simulink model "QET_KV"  (R2015b)
settings: Solver=ode4  SolverMode=SingleTasking  StartTime=0.0  StopTime=inf  FixedStep=Ts  RelTol=1e-3
values from neighbouring files (symbols this model uses):
  F_M_Direction = [1 1 1 -1 -1 -1]    [Config_StepperMotor.m]
  NanoCal7342 = [-0.945276141167 14.673559188843 0.251662999392 -14.892200469971 -0.854624807835 0.034513175488 ... (first row only)    [NanoCalibration.m]
  Resolution = (360/200 * 1/64)    (= 0.028125)    [Config_StepperMotor.m]
undefined symbols (not defined in the file or in its folder): AnalogPos_to_deg, anVE, anVE_GBC_Kbi, anVE_GBC_Kbp, anVE_K_int, anVE_Position_Gain_inv, anVE_Saturation, B, Chirp_Amplitude, Chirp_Freq_Max, Chirp_Freq_Min, Chirp_Period, Chirp_Time_Start, Chirp_Type, delay, Delta, DO_DG409_A0, DO_DG409_A1, Driver_Type, HIL, K, K_gyro, Kd, Kp, lambda, mag, Pos_Final, Pos_Init, Pos_Threshold, PSoC_Freq, qc_get_step_size, Stabilization_Period, Test_type, Times, Torque_Threshold, Ts, Ts_loop, VE_Platform, VE_Type
libraries: quarc_library x22, simulink x13, dspsigops x1
(part 3 of 3)

== matlab function QET_KV/Stability Check and Control/Initial and Final Condition Control/MATLAB Function ==
  data: sw output; sw_Sequence output; Clock input; Times input; Pos_Init input; Pos_out output; Pos_in input; is_stable input; Pos_Final input
function [sw,sw_Sequence,Pos_out] = fcn(Clock,Times,Pos_Init,Pos_in,is_stable,Pos_Final)
%#codegen


sw = 1;
Pos_out = 0;

%%
% Starting Up
if (Clock<Times(1))
    sw = 1;
    sw_Sequence = 1;
    Pos_out = 0;
% Initial Condition
elseif (Clock<Times(2))
    sw = 1;
    sw_Sequence = 2;
    Pos_out = Pos_Init;
% Stability Test
elseif (Clock<Times(3))&&(is_stable)
    sw = 2;
    sw_Sequence = 3;
    %Pos_out = Pos_in;
    Pos_out = Pos_Final;
% Final Condition
else
    sw = 1;
    sw_Sequence = 4;
    Pos_out = Pos_Final;
end

== matlab function QET_KV/PSoC Comm/MATLAB Function1 ==
  data: K input; X input; cmd output uint8; clock input; en output
function [cmd, en] = fcn(K,X,clock)
%#codegen


%cmd = cast('     ','uint8');
sum_ = 0;
cmd = uint8(zeros(1,6));
if (clock == 0.5)
    en = 1;
%    cmd = cast('Kabcd','uint8');
    cmd(1) = uint8('K');
    cmd(2:5) = typecast(single(K),'uint8');
    
    sum_ = mod(sum(cmd),256);
    cmd(6) = 255-sum_;
    
elseif (clock == 1)
    en = 1;
    cmd(1) = uint8('X');
    cmd(2:5) = typecast(single(X),'uint8');
    
    sum_ = mod(sum(cmd),256);
    cmd(6) = 255-sum_;
elseif (clock == 4)
    en = 1;
    cmd(1) = uint8('X');
    cmd(2:5) = typecast(single(0),'uint8');
    
    sum_ = mod(sum(cmd),256);
    cmd(6) = 255-sum_;
else
    en = 0;
end

== matlab function QET_KV/Stability Check and Control/Stability Check/MATLAB Function ==
  data: is_stable output; Clock input; Times input; Pos input; Pos_LPF input; Pos_Init input; Stop_PosThreshold input; stop_sim output; stop_sim_final output; Torque_Threshold input; Torque_LPF input; Pos_Threshold input; Pos_Random input; Stab_Period input; is_saturated input
function [is_stable,stop_sim,stop_sim_final]   = fcn(Clock, Times, Pos, Pos_LPF, Pos_Init, Stop_PosThreshold, Torque_Threshold, Torque_LPF, Pos_Threshold, Pos_Random,Stab_Period,is_saturated)
%#codegen
%% Initialization
persistent var_is_stable clock_stop;
if isempty(var_is_stable)
    var_is_stable = 1;
end
if isempty(clock_stop)
    clock_stop = 10;
end
%Pos_Threshold = Pos_Init * 1.25;

%% Define if is NOT stable

%Based on position threshold during uncoupled test
%Between times(1) and times (3)
%if ((Clock >= Times(2))...
    %&&(Clock < Times(3))...
if ((Clock >= Times(1))...
    &&(abs(Pos) >= Pos_Threshold)...
    &&(var_is_stable==1))
    var_is_stable = 0;
    clock_stop = Clock+Stab_Period;
end

%Based on Torque Threshold
if ((Clock>=Times(1))...
    &&(Torque_LPF >= Torque_Threshold)...
    &&(var_is_stable==1))
    var_is_stable = 0;
    clock_stop = Clock+Stab_Period;
end

%If there is saturation
if ((Clock>=Times(1))...
    &&(is_saturated > 0.5)...
    &&(var_is_stable==1))
    var_is_stable = 0;
    clock_stop = Clock+Stab_Period;
end

%% Stop simulation rules
stop_sim = 0;

if (var_is_stable==1)
    if (Clock<Times(3))
        Pos_Abs_Error = abs(Pos_LPF - 0);
    else
        Pos_Abs_Error = abs(Pos_LPF - Pos_Random)*.75;
    end
else
    Pos_Abs_Error = abs(Pos_LPF - Pos_Random)*.75;
end

% If it is Stable
if ((var_is_stable == 1)...
    &&(Clock>Times(3)+1.5)...
    &&(Pos_Abs_Error <= Stop_PosThreshold))
    stop_sim = 1;
end 

% If it is NOT Stable
if ((var_is_stable == 0)...
    &&(Clock>clock_stop)...
    &&(Pos_Abs_Error <= Stop_PosThreshold))
    stop_sim = 1;
end 

%% Stop simulation based on final time
stop_sim_final = 0;
%if ((stop_sim == 0)&&(Clock >= Times(4)))
if (Clock >= Times(4))
    stop_sim_final = 1;
end

%%

is_stable = var_is_stable;

== matlab function QET_KV/PSoC Comm/MATLAB Function2 ==
  data: SW_Seq input; Is_Stable input; C output
function C  = fcn(SW_Seq,Is_Stable)
%#codegen


if ((SW_Seq <= 1)&&(Is_Stable))
    C = 5; % Do nothing
elseif ((SW_Seq <= 3)&&(Is_Stable))
    C = 1; % Start Init and Test
else
    C = 3; % Stop Test
end

== matlab function QET_KV/Chirp and White Noise/Chirp 1/MATLAB Function ==
  data: type input; clock input; y output; chirp_period input; chirp_start input; chirp_amp input; fmin input; fmax input; f output
function [y,f] = fcn(type,clock,...
                     chirp_period,chirp_start,...
                     chirp_amp,fmin,fmax)
%#codegen

%% Chirp rates




%%
if (clock <= chirp_start)
    t = 0;
elseif (clock < (chirp_start+chirp_period))
    t = clock-chirp_start;
else
    t = chirp_period;
end

switch(type)
    case 2 % Quadratic
        c_quad = (fmax-fmin)/chirp_period^2;
        f      = c_quad*t^2 + fmin;
        f_int  = c_quad/3 * t^3 + fmin*t;

    case 3 % Exponential
        c_exp       = (fmax/fmin)^(1/chirp_period);
        f      = fmin * c_exp^t;
        f_int  = fmin * ((c_exp^t - 1)/log(c_exp));
        
    otherwise % Linear
        c_linear    = (fmax-fmin)/chirp_period;
        f      = c_linear*t + fmin;
        f_int  = c_linear/2 * t^2 + fmin*t;
end

%% Output
y = chirp_amp*sin(2*pi*f_int);

== matlab function QET_KV/Chirp and White Noise/MATLAB Function1 ==
  data: Chirp_Amp input; K input; y output
function y = fcn(Chirp_Amp,K)
%#codegen

% For K = 0.3 and Chirp_Amp=1 provides 
% max angular position of around 20 deg.
K_ref = 0.3;

if (K >= K_ref)
   y = Chirp_Amp;% = 1;
else
   % Tries to avoid high position by reducing excitation.
   y = Chirp_Amp * (K/K_ref);
end

== matlab function QET_KV/Stability Check and Control/Stability Check/MATLAB Function1 ==
  data: is_stable output; Clock input; Times input; Pos input; Pos_LPF input; Pos_Init input; stop_sim output; stop_sim_final output
function [is_stable,stop_sim,stop_sim_final]   = fcn(Clock, Times, Pos, Pos_LPF, Pos_Init)
%#codegen
%% Initialization
persistent var_is_stable clock_stop;
if isempty(var_is_stable)
    var_is_stable = 1;
end
if isempty(clock_stop)
    clock_stop = 10;
end
Pos_Threshold = Pos_Init * 1.25;

%% Code
if (Clock>=Times(2))&&(abs(Pos) >= Pos_Threshold)&&(var_is_stable==1)
    var_is_stable = 0;
    clock_stop = Clock+2;
end

if (var_is_stable == 0)&&(Clock>clock_stop)&&(Pos_LPF <= 0.02*Pos_Init)
    stop_sim = 1;
else
    stop_sim = 0;
end 

if (var_is_stable == 1)&&(Clock>Times(3)+1)&&(Pos_LPF <= 0.02*Pos_Init)
    stop_sim = 1;
else
    stop_sim = 0;
end 

stop_sim_final = 0;
%if ((stop_sim == 0)&&(Clock >= Times(4)))
if (Clock >= Times(4))
    stop_sim_final = 1;
end


is_stable = var_is_stable;

== matlab function QET_KV/Stability Check and Control/Initial and Final Condition Control/MATLAB Function1 ==
  data: QET_Pos input; Pos_Final input; DesiredPos input; INT_Enc input; Pos_Final_out output
function Pos_Final_out = fcn(QET_Pos,Pos_Final,DesiredPos,INT_Enc)
%#codegen

persistent Pos_Index;
if isempty(Pos_Index)
    Pos_Index = 0;
end

if((INT_Enc > 0)&&(Pos_Index == 0))
    Pos_Index = QET_Pos;
end

if (Pos_Index ~= 0)
    Pos_Final_out = Pos_Index+DesiredPos;
else
    Pos_Final_out = Pos_Final;
end

== matlab function QET_KV/Chirp and White Noise/MATLAB Function ==
  data: clock input; Gain_out output; Extra_Damping output; Chirp_Time_Start input; Gain_start input; Gain_in input; Torque_Excitation input; Torque_Haptic input; Saturation input; Torque_Rate output
function [Gain_out,Extra_Damping,Torque_Rate]   = fcn(clock,Chirp_Time_Start,...
                     Gain_start,Gain_in,...
                     Torque_Excitation,Torque_Haptic,...
                     Saturation)

%% Initialization
if (clock <= Chirp_Time_Start)
    Gain_out = Gain_start;
else
    Gain_out = Gain_in;    
end

%% 

Torque_Sum = Torque_Excitation + Torque_Haptic;
if (Torque_Sum>0)
    Torque_Rate = Torque_Excitation/Torque_Sum;
else
    Torque_Rate = 0;
end

if (Torque_Rate > 0.4)
	Extra_Damping = 0;
else
    % This means VE torque is increasing too much
    % Will lead to instability
    % Some damping is added to excitation signal
    Extra_Damping = 1; 
end

%% Saturation
if (Gain_out > Saturation(1))
    Gain_out = Saturation(1);
elseif (Gain_out < Saturation(2))
    Gain_out = Saturation(2);
end

== matlab function QET_KV/Stepper Motor/Stepper Motor Control Absolute/MATLAB Function ==
  data: PWM output; Pos_Ref input; Pos_Counter input; Pos_Enc_Deg input; Pos_Select input; DIR output; ENA output; Pos_out output; Resolution input; e output; Kp input; Clock input; Res_Bias output
function [PWM,DIR,ENA,Pos_out,e,Res_Bias] = fcn(Pos_Ref,Pos_Counter,Pos_Enc_Deg,Pos_Select,Resolution,Kp, Clock)
% function [DIR,Pos_out,Ref_out] = fcn(Pulse_new)

%% Initialization
persistent Pos_Ideal DIR_per PWM_old Pos_enc_error Res_Bias_per;
if isempty(Pos_Ideal)
    Pos_Ideal = 0; DIR_per = 0; PWM_old = 0; Pos_enc_error = 0;
    Res_Bias_per = 1;
end

%% Select Position Source
% Pos_Select = 1; %% 2 = Pos_Enc | 1 = Counter Input | 0 = Ideal Integration

if (Pos_Select == 2)
    if ((abs(Pos_Enc_Deg - (Pos_Counter * Resolution)) > 5)||(Pos_enc_error))
        Pos_enc_error = 1;
        Pos_Pulses = Pos_Counter;
        Pos = Pos_Counter * Resolution;
    else
        Pos = Pos_Enc_Deg;
    end
elseif (Pos_Select == 1)
    Pos_Pulses = Pos_Counter;
    Pos = Pos_Counter * Resolution;
else
    Pos_Pulses = round(Pos_Ideal / Resolution);
    Pos = Pos_Ideal;
end

%% Command
fmin = 1; % Minimum PWM frequency as Full Step [Hz]
fmax = 1000; % Maximum PWM frequency as Full Step [Hz]

fmin = fmin * (1/(Resolution * 200/360));
fmax = fmax * (1/(Resolution * 200/360));

Ts = 0.001;
Ts_R = 0.001 * Resolution;

Pos_Ref_Pulses = round(Pos_Ref / Resolution);

% e_pulses = abs(Pos_Ref_Pulses - Pos_Pulses); % [Pulses]

e = abs(Pos_Ref - Pos); % [Deg]

Res_Bias = Res_Bias_per;
%     if (Pos_Ref_Pulses - Pos_Pulses > 0) % Direction
if (Pos_Ref - Pos > 0) % Direction
    if (DIR_per == 0)
        Res_Bias = 3; Res_Bias_per = Res_Bias;
    end
    DIR_per = 1;
    DIR = DIR_per;
else
    if (DIR_per == 1)
        Res_Bias = 3; Res_Bias_per = Res_Bias;
    end
    DIR_per = 0;
    DIR = DIR_per;
end

if (e <= Resolution*Res_Bias)
    DIR = DIR_per;
    PWM = 0;
else
    Res_Bias = 1; Res_Bias_per = Res_Bias;
    
    % PWM_ = 5 * e_pulses * (1/(Resolution * 200/360)); % (1/(Resolution * 200/360)) = Micro-step compensation
    PWM_ = (e / Resolution) * Kp/Ts;

    PWM_ = round(PWM_/50)*50;

    if (PWM_ < fmin)
        PWM_ = fmin;
    elseif (PWM_ > fmax)
        PWM_ = fmax;
    end

    PWM_rate = (PWM_ - PWM_old)/Ts;
    if (PWM_rate > 1000)
        PWM_ = PWM_old + 1000;
    end

%     PWM = fmin;
    PWM_old = PWM_;
    PWM = PWM_;
end

%% Position Integration Based on Pulses (Ideal)
if (DIR > 0) % Direction
    Pos_Ideal = Pos_Ideal + PWM * Ts_R;
else
    Pos_Ideal = Pos_Ideal - PWM * Ts_R;
end
% Pos_Ideal = Pos_Ideal + 0.1;
%%
if (Pos_Select >= 1)
    Pos_out = Pos_Counter * Resolution;
else
    Pos_out = Pos_Ideal;
end


%% Initializing Driver

if (Clock <= 0.01)
    ENA = 1;
    PWM = 0;
    DIR_per = 0; DIR = DIR_per;
elseif (Clock <= 0.012)
    ENA = 0;
    PWM = 0.5/Ts * 0;
    DIR_per = 0; DIR = DIR_per;
elseif (Clock <= 0.014)
    ENA = 0;
    PWM = 0.5/Ts * 0;
    DIR_per = 1; DIR = DIR_per;
elseif (Clock <= 0.016)
    ENA = 0;
    PWM = 0.5/Ts * 0;
    DIR_per = 0; DIR = DIR_per;
elseif (Clock <= 0.018)
    ENA = 0;
    PWM = 0;
    DIR_per = 1; DIR = DIR_per;
else
    ENA = 0;
end

== matlab function QET_KV/Stepper Motor/Stepper Motor Control Absolute/MATLAB Function1 ==
  data: PWM output; Pos_Ref input; Pos_Counter input; Pos_Enc_Deg input; Pos_Select input; DIR output; Pos_out output; Resolution input; e output; Kp input; Clock input
function [PWM,DIR,Pos_out,e] = fcn(Pos_Ref,Pos_Counter,Pos_Enc_Deg,Pos_Select,Resolution,Kp, Clock)
% function [DIR,Pos_out,Ref_out] = fcn(Pulse_new)

%% Initialization
persistent Pos_Ideal DIR_per PWM_old Pos_enc_error;
if isempty(Pos_Ideal)
    Pos_Ideal = 0; DIR_per = 0; PWM_old = 0; Pos_enc_error = 0;
end

%% Select Position Source
% Pos_Select = 1; %% 2 = Pos_Enc | 1 = Counter Input | 0 = Ideal Integration

if (Pos_Select == 2)
    if ((abs(Pos_Enc_Deg - (Pos_Counter * Resolution)) > 5)||(Pos_enc_error))
        Pos_enc_error = 1;
        Pos_Pulses = Pos_Counter;
        Pos = Pos_Counter * Resolution;
    else
        Pos = Pos_Enc_Deg;
    end
elseif (Pos_Select == 1)
    Pos_Pulses = Pos_Counter;
    Pos = Pos_Counter * Resolution;
else
    Pos_Pulses = round(Pos_Ideal / Resolution);
    Pos = Pos_Ideal;
end

%% Command
fmin = 1; % Minimum PWM frequency as Full Step [Hz]
fmax = 1000; % Maximum PWM frequency as Full Step [Hz]

fmin = fmin * (1/(Resolution * 200/360));
fmax = fmax * (1/(Resolution * 200/360));

Ts = 0.001;
Ts_R = 0.001 * Resolution;

Pos_Ref_Pulses = round(Pos_Ref / Resolution);

% e_pulses = abs(Pos_Ref_Pulses - Pos_Pulses); % [Pulses]

e = abs(Pos_Ref - Pos); % [Deg]

if (e <= Resolution)
    DIR = DIR_per;
    PWM = 0;
else
%     if (Pos_Ref_Pulses - Pos_Pulses > 0) % Direction
    if (Pos_Ref - Pos > 0) % Direction
        DIR_per = 1;
        DIR = DIR_per;
    else
        DIR_per = 0;
        DIR = DIR_per;
    end

    % PWM_ = 5 * e_pulses * (1/(Resolution * 200/360)); % (1/(Resolution * 200/360)) = Micro-step compensation
    PWM_ = (e / Resolution) * Kp/Ts;

    PWM_ = round(PWM_/50)*50;

    if (PWM_ < fmin)
        PWM_ = fmin;
    elseif (PWM_ > fmax)
        PWM_ = fmax;
    end

    PWM_rate = (PWM_ - PWM_old)/Ts;
    if (PWM_rate > 1000)
        PWM_ = PWM_old + 1000;
    end

%     PWM = fmin;
    PWM_old = PWM_;
    PWM = PWM_;
end

%% Position Integration Based on Pulses (Ideal)
if (DIR > 0) % Direction
    Pos_Ideal = Pos_Ideal + PWM * Ts_R;
else
    Pos_Ideal = Pos_Ideal - PWM * Ts_R;
end
% Pos_Ideal = Pos_Ideal + 0.1;
%%
if (Pos_Select >= 1)
    Pos_out = Pos_Counter * Resolution;
else
    Pos_out = Pos_Ideal;
end


%% Initializing Driver

if (Clock <= 0.01)
    PWM = 0;
    DIR_per = 0;
    DIR = DIR_per;
elseif (Clock <= 0.012)
    PWM = 0.5/Ts;
    DIR_per = 0;
    DIR = DIR_per;
elseif (Clock <= 0.014)
    PWM = 0.5/Ts;
    DIR_per = 1;
    DIR = DIR_per;
elseif (Clock <= 0.016)
    PWM = 0.5/Ts;
    DIR_per = 0;
    DIR = DIR_per;
elseif (Clock <= 0.018)
    PWM = 0;
    DIR_per = 1;
    DIR = DIR_per;
end

== matlab function QET_KV/Chirp 2/MATLAB Function ==
  data: type input; clock input; y output; chirp_period input; chirp_start input; chirp_amp input; fmin input; fmax input; f output
function [y,f] = fcn(type,clock,...
                     chirp_period,chirp_start,chirp_amp,...
                     fmin,fmax)
%#codegen

%% Chirp rates




%%
if (clock <= chirp_start)
    t = 0;
elseif (clock < (chirp_start+chirp_period))
    t = clock-chirp_start;
else
    t = chirp_period;
end

switch(type)
    case 2 % Quadratic
        c_quad = (fmax-fmin)/chirp_period^2;
        f      = c_quad*t^2 + fmin;
        f_int  = c_quad/3 * t^3 + fmin*t;

    case 3 % Exponential
        c_exp       = (fmax/fmin)^(1/chirp_period);
        f      = fmin * c_exp^t;
        f_int  = fmin * ((c_exp^t - 1)/log(c_exp));
        
    otherwise % Linear
        c_linear    = (fmax-fmin)/chirp_period;
        f      = c_linear*t + fmin;
        f_int  = c_linear/2 * t^2 + fmin*t;
end

%% Output
y = chirp_amp*sin(2*pi*f_int);

== matlab function QET_KV/General Output/MATLAB Function ==
  data: override input; is_stable input; VE_Platform_Out output; VE_Platform input; VE_Platform_Manual input; DO output
function [VE_Platform_Out,DO] = fcn(override,is_stable,VE_Platform,VE_Platform_Manual)
%#codegen


%%
if (override >= 0.5)
    VE_Platform_Out = VE_Platform_Manual;
else
    if (is_stable > 0.5)
        % IF is stable and analog pos not saturated
        VE_Platform_Out = VE_Platform;
    else
        VE_Platform_Out = 1; % Digital VE
    end
end

%% Switch the DG403 circuit
if (VE_Platform_Out == 2)
    DO = 1; % Analog VE (Normal Open)
else
    DO = 0; % Digital VE (Normal Closed)
end

== matlab function QET_KV/Analog VE/GBC Method/MATLAB Function ==
  data: Clock input; Reset output; Time input; is_stable_vec input
function Reset  = fcn(Clock, Time, is_stable_vec)
%#codegen


if (Clock <= Time)
   Reset = 0; % DO Reset (Normal Closed)
elseif (is_stable_vec >= 0.5) % Is stable
        Reset = 1; % DO NOT Reset (Normal Closed)
else
        Reset = 0; % DO Reset (Normal Closed)
end
